simulink model "power_svc_3ph6t_f1"  (R2019a)
settings: Solver=VariableStepAuto  StartTime=0.0  StopTime=0.3  FixedStep=Ts  MaxStep=Ts  RelTol=1e-4  AbsTol=1e-4
PreLoadFcn:
  | Ts=50e-6;
undefined symbols (not defined in the file): D1, lagging, pulse
libraries: powerlib x16, powerlib_meascontrol x2
settings Model: ExtModeTrigMode=oneshot  ExtModeArmWhenConnect=off  ExtModeAutoUpdateStatusClock=off  Creator=MathWorks  LastModifiedBy=Walter Sanchez
settings SolverCC: AutoScaleAbsTol=off  ShapePreserveControl=EnableAll  ZeroCrossControl=EnableAll
settings DataIOCC: SaveFormat=StructureWithTime  SignalLoggingSaveFormat=ModelDataLogs  SaveOutput=off  SignalLogging=off  DSMLogging=off  SaveTime=off  ReturnWorkspaceOutputs=off  SignalLoggingName=sigsOut
settings OptimizationCC: BooleanDataType=off  ExpressionDepthLimit=2147483647  InitFltsAndDblsToZero=on  EfficientMapNaN2IntZero=off  LifeSpan=inf
settings DebuggingCC: UnderspecifiedInitializationDetection=Classic  MergeDetectMultiDrivingBlocksExec=none  CheckExecutionContextPreStartOutputMsg=on  CheckExecutionContextRuntimeOutputMsg=on  SignalResolutionControl=TryResolveAllWithWarning  MultiTaskDSMMsg=warning  MultiTaskCondExecSysMsg=none  FcnCallInpInsideContextMsg=warning  AllowSymbolicDim=off  StateNameClashWarn=warning  SFUnexpectedBacktrackingDiag=warning  SFNoUnconditionalDefaultTransitionDiag=warning  SFExecutionAtInitializationDiag=none  ArithmeticOperatorsInVariantConditions=warning
settings HardwareCC: ProdBitPerPointer=32  ProdBitPerSizeT=32  ProdBitPerPtrDiffT=32  ProdLargestAtomicFloat=None  ProdIntDivRoundTo=Undefined  ProdEndianess=Unspecified  ProdWordSize=32  ProdHWDeviceType=32-bit Generic  TargetUnknown=on
settings ModelReferenceCC: PropagateSignalLabelsOutOfModel=off
settings SFSimCC: SimUseLocalCustomCode=off
settings RTWCC: RTWUseLocalCustomCode=off
settings CodeAppCC: StateflowObjectComments=on
settings GRTTargetCC: TargetLangStandard=C89/C90 (ANSI)  CombineOutputUpdateFcns=off  GRTInterface=on
settings ConfigComp: CovMetricSettings=dw  CovSaveCumulativeToWorkspaceVar=on  CovSaveSingleToWorkspaceVar=on  CovExternalEMLEnable=off  CovSFcnEnable=off
settings SimscapeCC: SimscapeNormalizeSystem=off

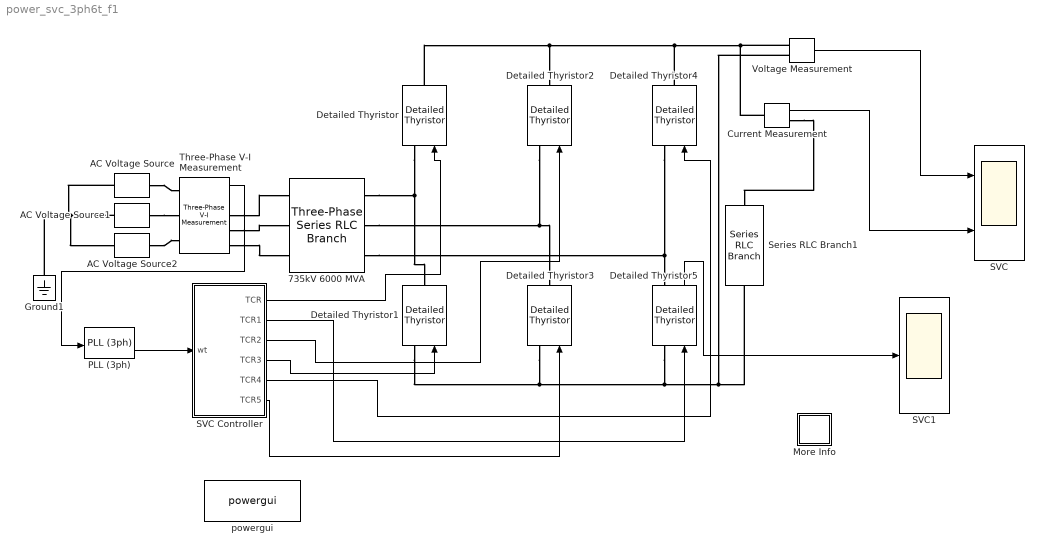
== system power_svc_3ph6t_f1 ==
  "735kV 6000 MVA " : powerlib/Elements/Three-Phase Series RLC Branch  LConnTagsString=A|B|C  RConnTagsString=A|B|C  BranchType=RL  Resistance=1.5  Inductance=1.0e-4  Capacitance=1.0  Measurements=None
  AC Voltage Source : powerlib/Electrical Sources/AC Voltage Source  Amplitude=179.6  Phase=0  Frequency=60  SampleTime=0  Measurements=Voltage  BusType=swing  Pref=10e3  Qref=0  Qmin=-inf  Qmax=+inf
  AC Voltage Source1 : powerlib/Electrical Sources/AC Voltage Source  Amplitude=179.6  Phase=120  Frequency=60  SampleTime=0  Measurements=Voltage  BusType=swing  Pref=10e3  Qref=0  Qmin=-inf  Qmax=+inf
  AC Voltage Source2 : powerlib/Electrical Sources/AC Voltage Source  Amplitude=179.6  Phase=240  Frequency=60  SampleTime=0  Measurements=Voltage  BusType=swing  Pref=10e3  Qref=0  Qmin=-inf  Qmax=+inf
  Current Measurement : powerlib/Measurements/Current Measurement  PhasorSimulation=off  OutputType=Complex  PSBequivalent=0
  Detailed Thyristor{,1..4} (5 alike) : powerlib/Power Electronics/Detailed Thyristor  Ron=0.001  Lon=1e-3  Vf=0.8  IL=0.1  Tq=100e-6  IC=0.01  Rs=500  Cs=250e-9  Measurements=off
      settings: SourceProductBaseCode=PS
  Detailed Thyristor5 : powerlib/Power Electronics/Detailed Thyristor  Ron=0.001  Lon=1e-3  Vf=0.8  IL=0.1  Tq=100e-6  IC=0.01  Rs=500  Cs=250e-9  Measurements=on
      settings: SourceProductBaseCode=PS
  Ground1 : powerlib/Elements/Ground  LConnTagsString=a
  More Info : Subsystem
      settings: OpenFcn=showdemo(bdroot(gcb))
      mask Display: disp('?')
  PLL (3ph) : powerlib_meascontrol/PLL/PLL (3ph)  Fmin=45  Par_Init=[0, 60]  ParK=[180, 3200, 1]  TcD=1e-4  MaxRateChangeFreq=12  FilterCutOffFreq=25  Ts=0  AGC=on
  SVC : Scope  NumInputPorts=2
  SVC Controller : Subsystem  mask(SVC Controller){OpMode=Voltage regulation, Vref=1.0, KpKi=[0 800], Xs=0.01, Bmin_max=[-1.04  3.23], Bref=2.5, Ts=Ts}
      mask prompts: OpMode "Operation mode"; Vref "Reference voltage (pu):"; KpKi "Regulator gains [ Kp  Ki ]:"; Xs "Droop (pu/100MVA):"; Bmin_max "Min. and max. primary susceptances [ Bind Bcap] (pu/100MVA):"; Bref "Susceptance Bref (pu/100MVA) (Var control mode):"; Ts "Sample time (s):"
      mask help:
      | This block implements a controller for a Static Var Compensator (SVC) consisting of one thyristor-controlled reactor bank (TCR) and three thyristor-switched capacitor banks (TSCs). Outputs TCR, TSC1, TSC2 and TSC3 are vectors of six pulses for the TCR and the three TSCs.
      | In Voltage control mode the primary voltage (Vabc_prim) is controlled at Vref within the maximum inductive and capacitive susceptance range and droop setting. In Var control mode the SVC susceptance  is  kept constant at Bref (Bref<0 for inductive mode).
      | Thyristor pulses are synchronized on secondary line-to-line voltages (Vabc_sec) of the coupling transformer, assuming a Wye/Delta (D1) connection.
      mask init:
      | Kp=KpKi(1);
      | Ki=KpKi(2);
      | Bmin=Bmin_max(1);
      | Bmax=Bmin_max(2);
      mask TypeOptions OpMode: Voltage regulation | Var control (Fixed susceptance Bref)
  SVC1 : Scope
  Series RLC Branch1 : powerlib/Elements/Series RLC Branch  LConnTagsString=__new0  RConnTagsString=__new0  BranchType=R  Resistance=10  Inductance=10e-3  SetiL0=off  InitialCurrent=0  Capacitance=1e-6  Setx0=off  InitialVoltage=0  Measurements=None
  Three-Phase V-I Measurement : powerlib/Measurements/Three-Phase V-I Measurement  VoltageMeasurement=phase-to-ground  SetLabelV=off  LabelV=Vabc  Vpu=off  VpuLL=off  CurrentMeasurement=yes  SetLabelI=off  LabelI=Iabc  Ipu=off  Pbase=100e6  Vbase=500e3  OutputType=Complex  PhasorSimulation=off  PSBequivalent=0
  Voltage Measurement : powerlib/Measurements/Voltage Measurement  PhasorSimulation=off  OutputType=Complex  PSBequivalent=0
  powergui : powerlib/powergui  Priority=2  SimulationMode=Continuous  SampleTime=Ts  frequency=60  Iterations=50  frequencyindice=60  Pbase=100e6  ErrMax=1e-4  UnitsV=kV  UnitsW=MW  buscounter=0  FunctionMessages=off  echomessages=off  EnableUseOfTLC=off  CurrentSourceSwitches=off  DisableSnubberDevices=off  DisableRonSwitches=off  DisableVfSwitches=off  DisplayEquations=off  AutomaticDiscreteSolvers=off  SolverType=Tustin/Backward Euler (TBE)  Interpol=off  ExternalGateDelay=off  methode=off  Ts=0  x0status=blocks  SPID=off  SwTol=0  HookPort=off  NonlinearTolerance=0  nMaxIteration=15  ContinueOnMaxIteration=off  RestoreLinks=warning  ResistiveCurrentMeasurement=off  Frange=[0:2:500]  Ylog=off  Xlog=on  ShowGrid=off  save=off  variable=ZData  structure=0  ZoomFFT=on  StartTime=0.0  cycles=1  DisplayStyle=1  fundamental=60  FreqAxis=off  MaxFrequency=1000  frequencyindicesteady=1  RmsSteady=2  display=off
  wires:
  Current Measurement/1 -> SVC/2
  Voltage Measurement/1 -> SVC/1
  SVC Controller/1(TCR) -> Detailed Thyristor/1
  SVC Controller/2(TCR1) -> Detailed Thyristor5/1
  SVC Controller/3(TCR2) -> Detailed Thyristor2/1
  SVC Controller/4(TCR3) -> Detailed Thyristor1/1
  SVC Controller/5(TCR4) -> Detailed Thyristor4/1
  SVC Controller/6(TCR5) -> Detailed Thyristor3/1
  Detailed Thyristor5/1 -> SVC1/1
  PLL (3ph)/2 -> SVC Controller/1(wt)
  Three-Phase V-I Measurement/1 -> PLL (3ph)/1
  connections:
  Detailed Thyristor1/LConn1 -- Detailed Thyristor3/LConn1 -- Detailed Thyristor5/LConn1 -- Series RLC Branch1/RConn1 -- Voltage Measurement/LConn2
  Current Measurement/RConn1 -- Series RLC Branch1/LConn1
  Detailed Thyristor/LConn1 -- "735kV 6000 MVA "/RConn1 -- Detailed Thyristor1/RConn1
  Detailed Thyristor2/LConn1 -- "735kV 6000 MVA "/RConn2 -- Detailed Thyristor3/RConn1
  Detailed Thyristor/RConn1 -- Detailed Thyristor4/RConn1 -- Voltage Measurement/LConn1 -- Current Measurement/LConn1 -- Detailed Thyristor2/RConn1
  Detailed Thyristor4/LConn1 -- "735kV 6000 MVA "/RConn3 -- Detailed Thyristor5/RConn1
  AC Voltage Source/LConn1 -- AC Voltage Source1/LConn1 -- AC Voltage Source2/LConn1 -- Ground1/LConn1
  AC Voltage Source/RConn1 -- Three-Phase V-I Measurement/LConn1
  AC Voltage Source1/RConn1 -- Three-Phase V-I Measurement/LConn2
  AC Voltage Source2/RConn1 -- Three-Phase V-I Measurement/LConn3
  Three-Phase V-I Measurement/RConn1 -- "735kV 6000 MVA "/LConn1
  Three-Phase V-I Measurement/RConn2 -- "735kV 6000 MVA "/LConn2
  Three-Phase V-I Measurement/RConn3 -- "735kV 6000 MVA "/LConn3

== system power_svc_3ph6t_f1/More Info ==

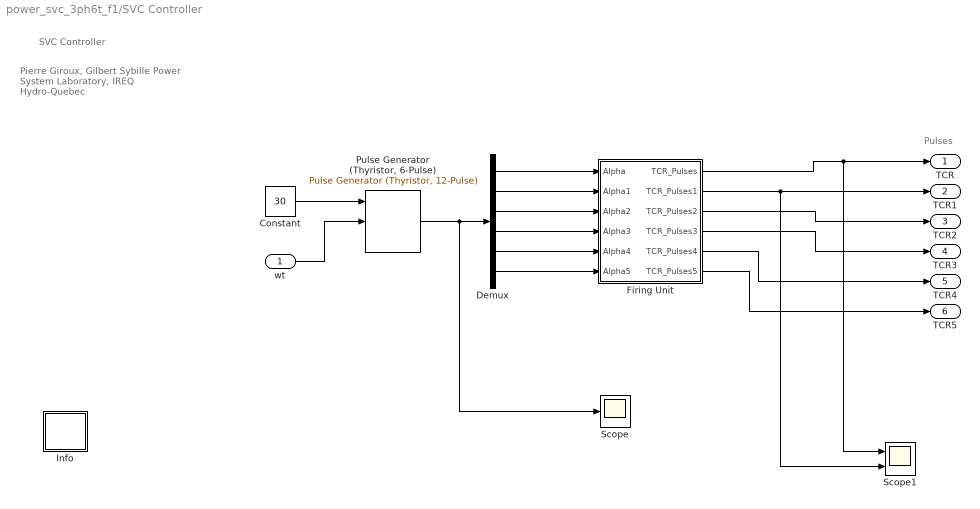
== system power_svc_3ph6t_f1/SVC Controller ==
  note: Pulses
  note: SVC Controller
  note: Pierre Giroux, Gilbert Sybille
      | Power System Laboratory, IREQ
      | Hydro-Quebec
  wt : Inport  PortDimensions=1
  Constant : Constant  Value=30
  Demux : Demux  Outputs=6
  Firing Unit : Subsystem  mask(Firing Unit){FiringMode=Continuous, Nstep=0, ParInit=[0 60], Ts=Ts}
      mask prompts: FiringMode "Firing mode"; Nstep "Total delay (in number of time step)"; ParInit "Initial phase and frequency of input: [ Phase (degree)  Freq (Hz) ]"; Ts "Sample time:"
      mask init:
      | PhaseInit=ParInit(1);
      | FreqInit=ParInit(2);
      mask TypeOptions FiringMode: Synchronized | Continuous
  Info : Subsystem
      mask Display: disp('?')
  "Pulse Generator (Thyristor, 6-Pulse)" : powerlib_meascontrol/Pulse & Signal Generators/Pulse Generator (Thyristor, 12-Pulse)  GenType=6-pulse  Delta=D1 (lagging)  pwidth=60  Double_Pulse=on  Ts=0
      settings: SourceProductBaseCode=PS
  Scope : Scope
  Scope1 : Scope  NumInputPorts=2
  TCR : Outport  VectorParamsAs1DForOutWhenUnconnected=off
  TCR1 : Outport  Port=2  VectorParamsAs1DForOutWhenUnconnected=off
  TCR2 : Outport  Port=3  VectorParamsAs1DForOutWhenUnconnected=off
  TCR3 : Outport  Port=4  VectorParamsAs1DForOutWhenUnconnected=off
  TCR4 : Outport  Port=5  VectorParamsAs1DForOutWhenUnconnected=off
  TCR5 : Outport  Port=6  VectorParamsAs1DForOutWhenUnconnected=off
  wires:
  Firing Unit/1(TCR_Pulses) -> Scope1/1, TCR/1
  Firing Unit/2(TCR_Pulses1) -> Scope1/2, TCR1/1
  "Pulse Generator (Thyristor, 6-Pulse)"/1 -> Scope/1, Demux/1
  Demux/1 -> Firing Unit/1(Alpha)
  Demux/2 -> Firing Unit/2(Alpha1)
  Demux/3 -> Firing Unit/3(Alpha2)
  Demux/4 -> Firing Unit/4(Alpha3)
  Demux/5 -> Firing Unit/5(Alpha4)
  Demux/6 -> Firing Unit/6(Alpha5)
  Firing Unit/3(TCR_Pulses2) -> TCR2/1
  Firing Unit/4(TCR_Pulses3) -> TCR3/1
  Firing Unit/5(TCR_Pulses4) -> TCR4/1
  Firing Unit/6(TCR_Pulses5) -> TCR5/1
  Constant/1 -> "Pulse Generator (Thyristor, 6-Pulse)"/1
  wt/1 -> "Pulse Generator (Thyristor, 6-Pulse)"/2

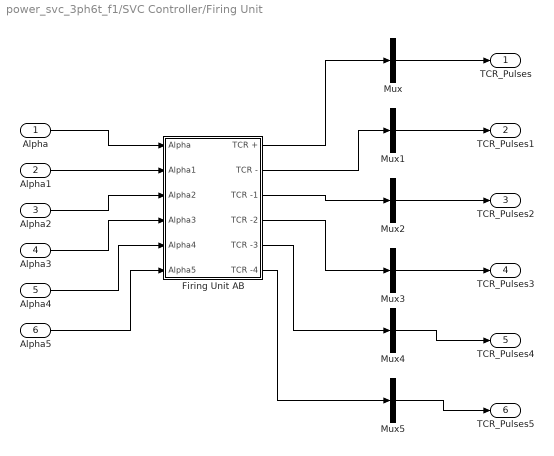
== system power_svc_3ph6t_f1/SVC Controller/Firing Unit ==
  Alpha : Inport  PortDimensions=1
  Alpha1 : Inport  Port=2  PortDimensions=1
  Alpha2 : Inport  Port=3  PortDimensions=1
  Alpha3 : Inport  Port=4  PortDimensions=1
  Alpha4 : Inport  Port=5  PortDimensions=1
  Alpha5 : Inport  Port=6  PortDimensions=1
  Firing Unit AB : Subsystem  mask{FiringMode=FiringMode, Nstep=Nstep, ParInit=[PhaseInit FreqInit], Ts=Ts}
      mask prompts: FiringMode "Firing Mode (1=Synchronized, 2=Continuous)"; Nstep "Total delay (in number of time step)"; ParInit "Initial phase and frequency of input: [ Phase (degree)  Freq (Hz) ]"; Ts "Sample time:"
      mask init:
      | PhaseInit=ParInit(1);
      | FreqInit=ParInit(2);
  Mux{,1..5} (6 alike) : Mux  Inputs=1
  TCR_Pulses : Outport  VectorParamsAs1DForOutWhenUnconnected=off
  TCR_Pulses1 : Outport  Port=2  VectorParamsAs1DForOutWhenUnconnected=off
  TCR_Pulses2 : Outport  Port=3  VectorParamsAs1DForOutWhenUnconnected=off
  TCR_Pulses3 : Outport  Port=4  VectorParamsAs1DForOutWhenUnconnected=off
  TCR_Pulses4 : Outport  Port=5  VectorParamsAs1DForOutWhenUnconnected=off
  TCR_Pulses5 : Outport  Port=6  VectorParamsAs1DForOutWhenUnconnected=off
  wires:
  Alpha/1 -> Firing Unit AB/1(Alpha)
  Firing Unit AB/1(TCR +) -> Mux/1
  Mux/1 -> TCR_Pulses/1
  Firing Unit AB/2(TCR -) -> Mux1/1
  Mux1/1 -> TCR_Pulses1/1
  Alpha1/1 -> Firing Unit AB/2(Alpha1)
  Mux2/1 -> TCR_Pulses2/1
  Firing Unit AB/3(TCR -1) -> Mux2/1
  Mux3/1 -> TCR_Pulses3/1
  Firing Unit AB/4(TCR -2) -> Mux3/1
  Mux4/1 -> TCR_Pulses4/1
  Mux5/1 -> TCR_Pulses5/1
  Firing Unit AB/5(TCR -3) -> Mux4/1
  Firing Unit AB/6(TCR -4) -> Mux5/1
  Alpha2/1 -> Firing Unit AB/3(Alpha2)
  Alpha3/1 -> Firing Unit AB/4(Alpha3)
  Alpha4/1 -> Firing Unit AB/5(Alpha4)
  Alpha5/1 -> Firing Unit AB/6(Alpha5)

== system power_svc_3ph6t_f1/SVC Controller/Info ==
  note: 1) Open-loop time constant evaluation:
  note: Xs -> Slope in pu/100MVA
      |  Ki -> Integral gain (puB/puV/s)
  note: where:
  note: Closed-loop time constant --> Tc ~= [ Xs / ( Xr + Xs ) ] * To
  note: Open-loop time constant --> To ~= 1 / ( Ki * Xs )
  note: To verify the following formula, open the loop (using the manual switch) and
      | add a 0.008 pu step to the reference voltage (Vref)
  note: 2) Misfiring simulation:
  note: To simulate a misfiring of thyristor AB+ of TSC1:
      | First switch off the TSC1 branch by adding a -0.008 pu to Vref at 0.04s
      | and then generate a firing pulse at 0.105s (one time step duration) using the Timer block

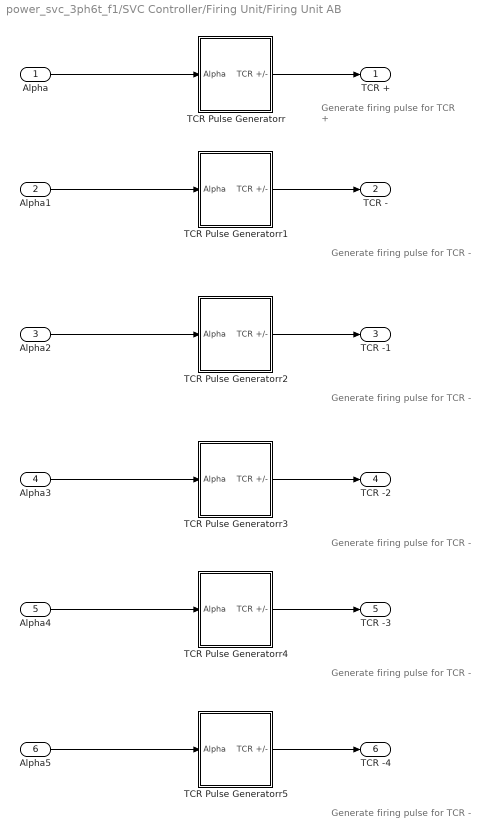
== system power_svc_3ph6t_f1/SVC Controller/Firing Unit/Firing Unit AB ==
  note: Generate firing
      | pulse for TCR +
  note: Generate firing
      | pulse for TCR -
  note: Generate firing
      | pulse for TCR -
  note: Generate firing
      | pulse for TCR -
  note: Generate firing
      | pulse for TCR -
  note: Generate firing
      | pulse for TCR -
  Alpha : Inport  PortDimensions=1
  Alpha1 : Inport  Port=2  PortDimensions=1
  Alpha2 : Inport  Port=3  PortDimensions=1
  Alpha3 : Inport  Port=4  PortDimensions=1
  Alpha4 : Inport  Port=5  PortDimensions=1
  Alpha5 : Inport  Port=6  PortDimensions=1
  TCR Pulse Generatorr : Subsystem  mask{Ts=Ts}
      mask prompts: Ts "Sample time:"
  TCR Pulse Generatorr1 : Subsystem  mask{Ts=Ts}
      mask prompts: Ts "Sample time:"
  TCR Pulse Generatorr2 : Subsystem  mask{Ts=Ts}
      mask prompts: Ts "Sample time:"
  TCR Pulse Generatorr3 : Subsystem  mask{Ts=Ts}
      mask prompts: Ts "Sample time:"
  TCR Pulse Generatorr4 : Subsystem  mask{Ts=Ts}
      mask prompts: Ts "Sample time:"
  TCR Pulse Generatorr5 : Subsystem  mask{Ts=Ts}
      mask prompts: Ts "Sample time:"
  TCR + : Outport  VectorParamsAs1DForOutWhenUnconnected=off
  TCR - : Outport  Port=2  VectorParamsAs1DForOutWhenUnconnected=off
  TCR -1 : Outport  Port=3  VectorParamsAs1DForOutWhenUnconnected=off
  TCR -2 : Outport  Port=4  VectorParamsAs1DForOutWhenUnconnected=off
  TCR -3 : Outport  Port=5  VectorParamsAs1DForOutWhenUnconnected=off
  TCR -4 : Outport  Port=6  VectorParamsAs1DForOutWhenUnconnected=off
  wires:
  TCR Pulse Generatorr/1(TCR +/-) -> TCR +/1
  Alpha/1 -> TCR Pulse Generatorr/1(Alpha)
  TCR Pulse Generatorr1/1(TCR +/-) -> TCR -/1
  Alpha1/1 -> TCR Pulse Generatorr1/1(Alpha)
  TCR Pulse Generatorr2/1(TCR +/-) -> TCR -1/1
  Alpha2/1 -> TCR Pulse Generatorr2/1(Alpha)
  TCR Pulse Generatorr3/1(TCR +/-) -> TCR -2/1
  Alpha3/1 -> TCR Pulse Generatorr3/1(Alpha)
  TCR Pulse Generatorr4/1(TCR +/-) -> TCR -3/1
  Alpha4/1 -> TCR Pulse Generatorr4/1(Alpha)
  TCR Pulse Generatorr5/1(TCR +/-) -> TCR -4/1
  Alpha5/1 -> TCR Pulse Generatorr5/1(Alpha)

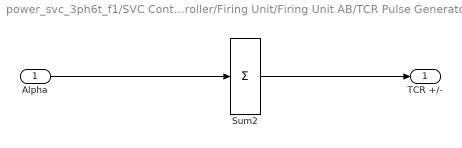
== system power_svc_3ph6t_f1/SVC Controller/Firing Unit/Firing Unit AB/TCR Pulse Generatorr ==
  Alpha : Inport  PortDimensions=1
  Sum2 : Sum  Inputs=+  InputSameDT=on  SaturateOnIntegerOverflow=on  OutDataTypeStr=Inherit: Same as first input
  TCR +/- : Outport  VectorParamsAs1DForOutWhenUnconnected=off
  wires:
  Sum2/1 -> TCR +/-/1
  Alpha/1 -> Sum2/1

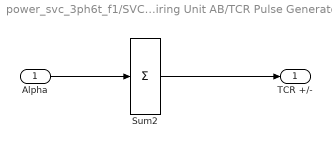
== system power_svc_3ph6t_f1/SVC Controller/Firing Unit/Firing Unit AB/TCR Pulse Generatorr1 ==
  Alpha : Inport  PortDimensions=1
  Sum2 : Sum  Inputs=+  InputSameDT=on  SaturateOnIntegerOverflow=on  OutDataTypeStr=Inherit: Same as first input
  TCR +/- : Outport  VectorParamsAs1DForOutWhenUnconnected=off
  wires:
  Alpha/1 -> Sum2/1
  Sum2/1 -> TCR +/-/1

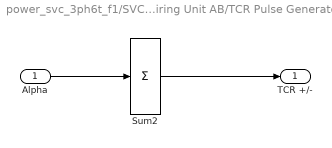
== system power_svc_3ph6t_f1/SVC Controller/Firing Unit/Firing Unit AB/TCR Pulse Generatorr2 ==
  Alpha : Inport  PortDimensions=1
  Sum2 : Sum  Inputs=+  InputSameDT=on  SaturateOnIntegerOverflow=on  OutDataTypeStr=Inherit: Same as first input
  TCR +/- : Outport  VectorParamsAs1DForOutWhenUnconnected=off
  wires:
  Alpha/1 -> Sum2/1
  Sum2/1 -> TCR +/-/1

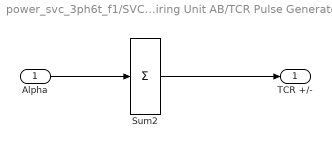
== system power_svc_3ph6t_f1/SVC Controller/Firing Unit/Firing Unit AB/TCR Pulse Generatorr3 ==
  Alpha : Inport  PortDimensions=1
  Sum2 : Sum  Inputs=+  InputSameDT=on  SaturateOnIntegerOverflow=on  OutDataTypeStr=Inherit: Same as first input
  TCR +/- : Outport  VectorParamsAs1DForOutWhenUnconnected=off
  wires:
  Alpha/1 -> Sum2/1
  Sum2/1 -> TCR +/-/1

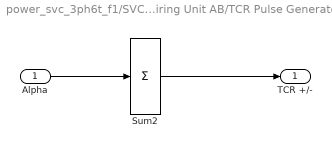
== system power_svc_3ph6t_f1/SVC Controller/Firing Unit/Firing Unit AB/TCR Pulse Generatorr4 ==
  Alpha : Inport  PortDimensions=1
  Sum2 : Sum  Inputs=+  InputSameDT=on  SaturateOnIntegerOverflow=on  OutDataTypeStr=Inherit: Same as first input
  TCR +/- : Outport  VectorParamsAs1DForOutWhenUnconnected=off
  wires:
  Alpha/1 -> Sum2/1
  Sum2/1 -> TCR +/-/1

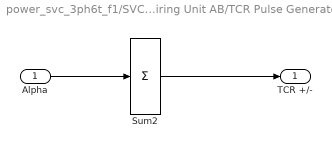
== system power_svc_3ph6t_f1/SVC Controller/Firing Unit/Firing Unit AB/TCR Pulse Generatorr5 ==
  Alpha : Inport  PortDimensions=1
  Sum2 : Sum  Inputs=+  InputSameDT=on  SaturateOnIntegerOverflow=on  OutDataTypeStr=Inherit: Same as first input
  TCR +/- : Outport  VectorParamsAs1DForOutWhenUnconnected=off
  wires:
  Alpha/1 -> Sum2/1
  Sum2/1 -> TCR +/-/1
